simulink model "lab2model"  (R2021a)
settings: Solver=VariableStepAuto  StartTime=0.0  StopTime=10.0  RelTol=1e-3
settings Model: Creator=ajendo  LastModifiedBy=adrian

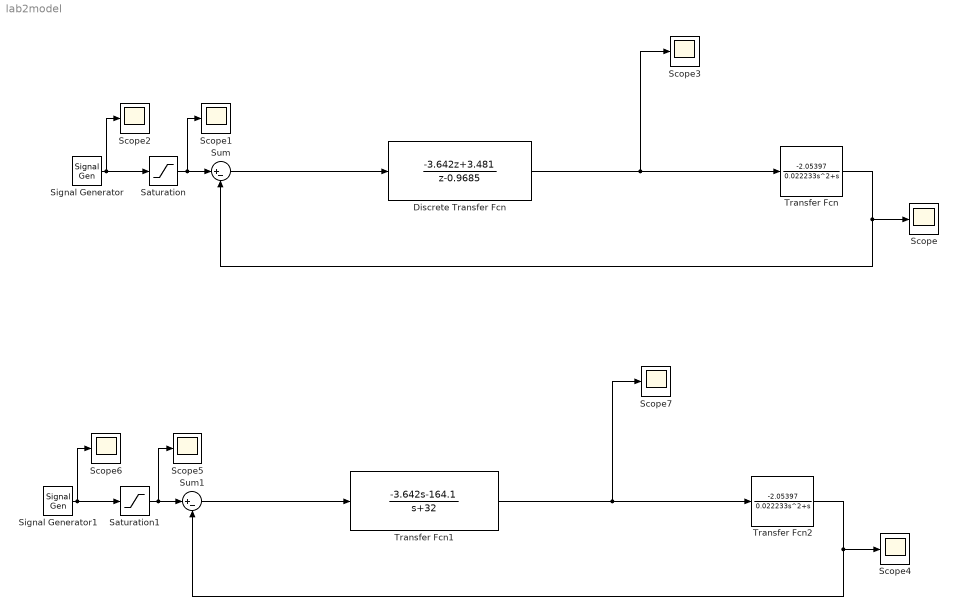
== system lab2model ==
  Discrete Transfer Fcn : DiscreteTransferFcn  Numerator=[-3.642 3.481]  Denominator=[1 -0.9685]  SampleTime=[0.001, 0]
  Saturation : Saturate  UpperLimit=0.7  LowerLimit=-0.7
  Saturation1 : Saturate  UpperLimit=0.7  LowerLimit=-0.7
  Scope{,1..7} (8 alike) : Scope
  Signal Generator : SignalGenerator  WaveForm=square  Amplitude=2  Units=rad/sec
  Signal Generator1 : SignalGenerator  WaveForm=square  Amplitude=2  Units=rad/sec
  Sum : Sum  Inputs=|+-
  Sum1 : Sum  Inputs=|+-
  Transfer Fcn : TransferFcn  Numerator=[-2.05397]  Denominator=[0.022233 1 0]
  Transfer Fcn1 : TransferFcn  Numerator=[-3.642 -164.1]  Denominator=[1 32]
  Transfer Fcn2 : TransferFcn  Numerator=[-2.05397]  Denominator=[0.022233 1 0]
  wires:
  Transfer Fcn/1 -> Sum/2, Scope/1
  Saturation/1 -> Scope1/1, Sum/1
  Signal Generator/1 -> Scope2/1, Saturation/1
  Discrete Transfer Fcn/1 -> Scope3/1, Transfer Fcn/1
  Sum/1 -> Discrete Transfer Fcn/1
  Transfer Fcn1/1 -> Scope7/1, Transfer Fcn2/1
  Sum1/1 -> Transfer Fcn1/1
  Signal Generator1/1 -> Scope6/1, Saturation1/1
  Transfer Fcn2/1 -> Sum1/2, Scope4/1
  Saturation1/1 -> Scope5/1, Sum1/1
